simulink model "Cintroller"  (R2020a)
settings: Solver=VariableStepAuto  StartTime=0.0  StopTime=1  RelTol=1e-3  EnableMultiTasking=on
settings Model: Creator=asuS  LastModifiedBy=Hossein
settings DataIOCC: LimitDataPoints=on  ReturnWorkspaceOutputs=off
settings OptimizationCC: LifeSpan=inf
settings DebuggingCC: AllowSymbolicDim=off  SFUnexpectedBacktrackingDiag=warning  SFNoUnconditionalDefaultTransitionDiag=warning  SFExecutionAtInitializationDiag=none  ArithmeticOperatorsInVariantConditions=warning
settings ModelReferenceCC: PropagateSignalLabelsOutOfModel=off
settings SFSimCC: SimUseLocalCustomCode=off  CustomCodeUndefinedFunction=UseInterfaceOnly
settings RTWCC: RTWUseLocalCustomCode=off
settings CodeAppCC: StateflowObjectComments=on
settings GRTTargetCC: TargetLangStandard=C89/C90 (ANSI)
settings ConfigComp: CovMetricSettings=dw  CovHtmlReporting=on  CovSaveCumulativeToWorkspaceVar=on  CovSaveSingleToWorkspaceVar=on  CovExternalEMLEnable=off

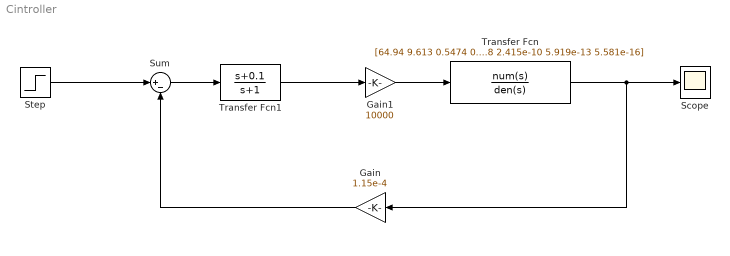
== system Cintroller ==
  Gain : Gain  Gain=1.15e-4
  Gain1 : Gain  Gain=10000
  Scope : Scope
  Step : Step  Time=0  After=3.4899e-5  SampleTime=0
  Sum : Sum  Inputs=|+-
  Transfer Fcn : TransferFcn  Numerator=[64.94 9.613 0.5474 0.01506 0.0002085 1.427e-6 4.358e-9 4.768e-12]  Denominator=[1 0.1595 0.009992 0.0003134 5.269e-6 4.864e-8 2.415e-10 5.919e-13 5.581e-16]
  Transfer Fcn1 : TransferFcn  Numerator=[1 0.1]  Denominator=[1 1]
  wires:
  Step/1 -> Sum/1
  Transfer Fcn/1 -> Gain/1, Scope/1
  Gain/1 -> Sum/2
  Sum/1 -> Transfer Fcn1/1
  Transfer Fcn1/1 -> Gain1/1
  Gain1/1 -> Transfer Fcn/1
